simulink model "mpc11"  (R2022b)
settings: Solver=ode4  StartTime=0.0  StopTime=10  FixedStep=0.001  RelTol=1e-3
undefined symbols (not defined in the file or in its folder): DiscIntNeverNeededParam
settings Model: Creator=hanli  LastModifiedBy=hanli
settings SolverCC: AlgebraicLoopSolver=TrustRegion
settings DebuggingCC: UnconnectedInputMsg=warning  UnconnectedOutputMsg=warning  UnconnectedLineMsg=warning  SFMachineParentedDataDiag=warning  UnderSpecifiedDimensionMsg=warning
settings ModelReferenceCC: EnableRefExpFcnMdlSchedulingChecks=on

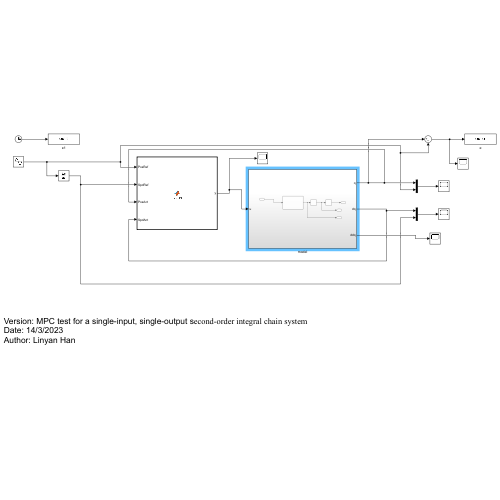
[thumbnail: Simulink's stored preview of the top-level diagram]
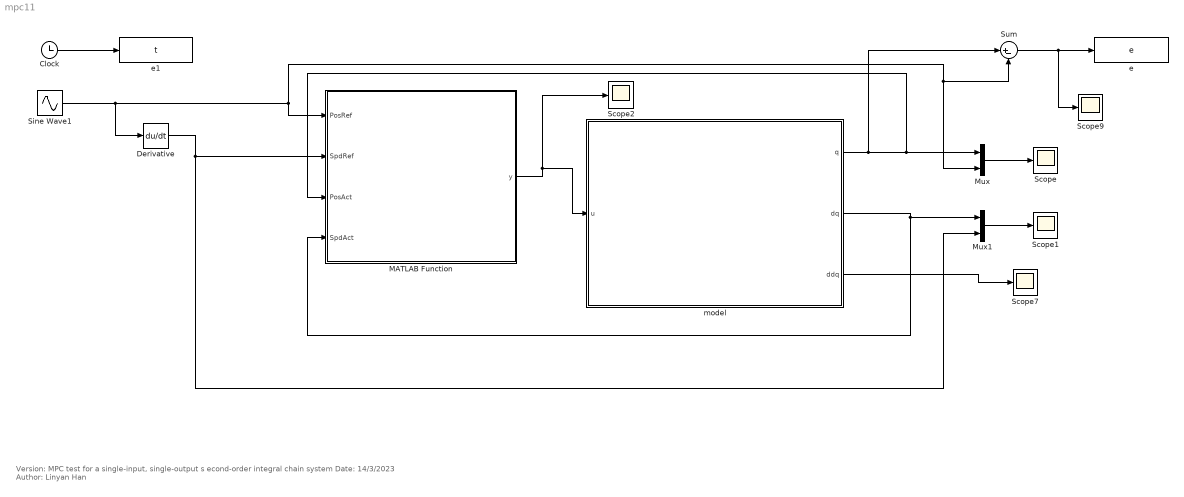
== system mpc11 ==
  note: Version: MPC test for a single-input, single-output s econd-order integral chain system
      | Date: 14/3/2023
      | Author: Linyan Han
  Clock : Clock
  Derivative : Derivative
  MATLAB Function : MATLAB Function  TreatAsAtomicUnit=on
  Mux : Mux  Inputs=2
  Mux1 : Mux  Inputs=2
  Scope{,1..2,7,9} (5 alike) : Scope
  Sine Wave1 : Sin  SampleTime=0
  Sum : Sum  Inputs=|+-
  e : ToWorkspace  VariableName=e  SampleTime=-1
  e1 : ToWorkspace  VariableName=t  SampleTime=-1
  model : Subsystem
  wires:
  Derivative/1 -> MATLAB Function/2(SpdRef), Mux1/2
  Mux/1 -> Scope/1
  MATLAB Function/1(y) -> model/1(u), Scope2/1
  Clock/1 -> e1/1
  Sum/1 -> Scope9/1, e/1
  Sine Wave1/1 -> Derivative/1, Sum/2, Mux/2, MATLAB Function/1(PosRef)
  model/1(q) -> Sum/1, Mux/1, MATLAB Function/3(PosAct)
  Mux1/1 -> Scope1/1
  model/3(ddq) -> Scope7/1
  model/2(dq) -> Mux1/1, MATLAB Function/4(SpdAct)

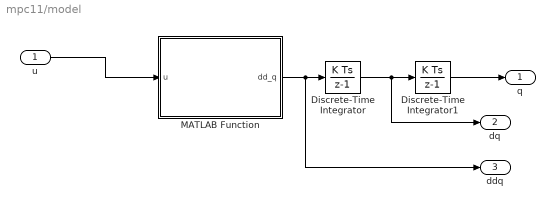
== system mpc11/model ==
  u : Inport
  Discrete-Time Integrator : DiscreteIntegrator  SampleTime=-1  ICPrevOutput=DiscIntNeverNeededParam  ICPrevScaledInput=DiscIntNeverNeededParam
  Discrete-Time Integrator1 : DiscreteIntegrator  SampleTime=-1  ICPrevOutput=DiscIntNeverNeededParam  ICPrevScaledInput=DiscIntNeverNeededParam
  MATLAB Function : MATLAB Function  TreatAsAtomicUnit=on
  q : Outport
  dq : Outport  Port=2
  ddq : Outport  Port=3
  wires:
  u/1 -> MATLAB Function/1(u)
  MATLAB Function/1(dd_q) -> Discrete-Time Integrator/1, ddq/1
  Discrete-Time Integrator/1 -> Discrete-Time Integrator1/1, dq/1
  Discrete-Time Integrator1/1 -> q/1

== matlab function mpc11/MATLAB Function ==
  settings: updateMethod=DISCRETE
  data: PosRef input; y output; SpdRef input; PosAct input; SpdAct input
function y =mpc11(PosRef,SpdRef,PosAct,SpdAct)

% %%%%%%%%%%%%%%%%%%%%%%%%%%%%
h1= 0.001;%采样时间
Ap = [1 h1;0 1];
Bp = [0;h1];   
Cp = [1 0];

rk=PosRef;
% % %%%%%%%%%%%% 初始化 %%%%%%%%%%%%%
Np=25;
Nc =1;
R =0.01*eye(Nc);
Q = 50000*eye(Np);
%%%%%%%%%%%%%%%%%%%%%%%%%%%%%%%%%%%% 

[m2,n2]=size(Cp);
h=zeros(Np,n2);
h(1,:)=Cp; 

[m3,n3]=size(Cp*Ap);
F=zeros(Np,n3);
F(1,:)=Cp*Ap;

[m4,n4]=size(Cp);
lc=zeros(Np,n4);
lc(1,:)=Cp;

[m5,n5]=size(Cp);
Phif=zeros(Np,n5);
Phif(1,:)=Cp;

for kk=2:Np
    h(kk,:)=h(kk-1,:)*Ap;
    F(kk,:)=F(kk-1,:)*Ap;
    Phif(kk,:)=Phif(kk-1,:)*Ap+Cp;
end

for kk=2:(Np-Nc+1)
    lc(kk,:)=lc(kk-1,:)*Ap+Cp;
end

v=h*Bp;
w=lc*Bp;
Phif = Phif*Bf;

Phi=zeros(Np,Nc);
Phi(:,1)=v;
for i=2:Nc-1
    Phi(:,i)=[zeros(i-1,1);v(1:Np-i+1,1)];
end

Phi(:,Nc)=[zeros(Nc-1,1);w(1:Np-Nc+1,1)];
BarRs = ones(Np,1)*rk;
Phi_Phi = Phi'*Q* Phi;
Phi_F = Phi'*Q* F;
Phi_R = Phi'*Q* BarRs;
Phi_Phif = Phi' *Q* Phif;
IPhi_Phif = pinv(Phi) * Phif;

xr= [PosRef;SpdRef];
est_u =  pinv(Phi)*(BarRs - F * xr );
 sigma = Phi_Phi + R;
 omega=R*est_u+Phi_R- Phi_F*[PosAct;SpdAct];
  
% %%%%%%%%% 无约束情况的控制律 %%%%%%%%%
% u_q = inv(sigma)*omega;
% y = u_q(1);

% %%%%%%%%% 有约束情况的控制律 %%%%%%%%%
theta = [1;-1;1;-1];
dq_min = -1;%速度约束
dq_max = 1;%
ddq_min = -10;%%加速度约束
ddq_max = 10;%
Theta = blkdiag(theta);%与Nc有关
gama = [(dq_max - SpdAct)/h1; -(dq_min - SpdAct)/h1; ddq_max; -ddq_min];
Gama = [gama];%与Nc有关
u_q = QPhild(sigma, -omega, Theta, Gama);%注意之前调试发散是因为omega的值差了一个负号引起的；
y = u_q(1);%与Nc有关，取第一项

== matlab function mpc11/model/MATLAB Function ==
  data: u input; dd_q output
function dd_q = f(u)

dd_q = u;
